simulink model "pend_dob_v"  (R2018b)
settings: Solver=VariableStepAuto  StartTime=0.0  StopTime=20  MaxStep=1e-2  RelTol=1e-3
values from neighbouring files (symbols this model uses):
  g = 9.8    [pendulo_circular.m]    (also in pendulo_doble.m; pendulo_giratorio.m)
  l1 = 0.25    [pendulo_doble.m]
  l2 = 0.5    [pendulo_doble.m]
  m1 = 0.5    [pendulo_doble.m]
  t1ini = deg2rad(10)    [pendulo_doble.m]
  t1pini = deg2rad(0)    [pendulo_doble.m]
  t2ini = deg2rad(60)    [pendulo_doble.m]
  t2pini = deg2rad(0)    [pendulo_doble.m]
settings Model: Creator=Acer  LastModifiedBy=Acer
settings DataIOCC: ReturnWorkspaceOutputs=on

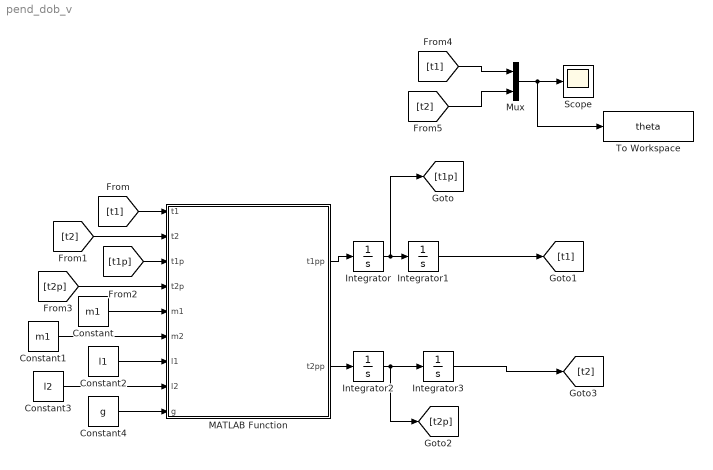
== system pend_dob_v ==
  Constant : Constant  Value=m1
  Constant1 : Constant  Value=m1
  Constant2 : Constant  Value=l1
  Constant3 : Constant  Value=l2
  Constant4 : Constant  Value=g
  Integrator : Integrator  InitialCondition=t1pini
  Integrator1 : Integrator  InitialCondition=t1ini
  Integrator2 : Integrator  InitialCondition=t2pini
  Integrator3 : Integrator  InitialCondition=t2ini
  MATLAB Function : MATLAB Function  TreatAsAtomicUnit=on
  Mux : Mux  Inputs=2
  Scope : Scope
  To Workspace : ToWorkspace  VariableName=theta  SaveFormat=Structure With Time  SampleTime=-1
  wires:
  MATLAB Function/1(t1pp) -> Integrator/1
  Integrator/1 -> [t1p], Integrator1/1
  MATLAB Function/2(t2pp) -> Integrator2/1
  Integrator2/1 -> Integrator3/1, [t2p]
  [t1] -> MATLAB Function/1(t1)
  Integrator1/1 -> [t1]
  [t2] -> MATLAB Function/2(t2)
  [t1p] -> MATLAB Function/3(t1p)
  [t2p] -> MATLAB Function/4(t2p)
  Integrator3/1 -> [t2]
  Mux/1 -> To Workspace/1, Scope/1
  [t1] -> Mux/1
  [t2] -> Mux/2
  Constant/1 -> MATLAB Function/5(m1)
  Constant1/1 -> MATLAB Function/6(m2)
  Constant2/1 -> MATLAB Function/7(l1)
  Constant3/1 -> MATLAB Function/8(l2)
  Constant4/1 -> MATLAB Function/9(g)

== matlab function pend_dob_v/MATLAB Function ==
  data: t1 input; t1pp output; t2 input; t1p input; t2p input; t2pp output; m1 input; m2 input; l1 input; l2 input; g input
function [t1pp,t2pp] = fcn(t1,t2,t1p,t2p,m1,m2,l1,l2,g)
% m1=1;
% m2=1;
% l1=1;
% l2=1;
% g=9.8;

dt=t1-t2;
mu=1+m1/m2;
m=m1/m2;

% t1pp=(g*(sin(t2)*cos(dt)-mu*sin(t1))-sin(dt)*(l2*t2p^2+l1*t1p^2*cos(dt)))/(l1*(mu-(cos(dt))^2));
% t2pp=(g*mu*(sin(t1)*cos(dt)-sin(t2))-sin(dt)*(mu*l1*t1p^2+l2*t2p^2*cos(dt)))/(l2*(mu-(cos(dt))^2));

t1pp=(cos(dt)*((g/l1)*sin(t2)-t1p^2*sin(dt))-(l2/l1)*((m+1)*(g/l2)*sin(t1)+t2p^2*sin(dt)))/(m+(sin(dt))^2);
t2pp=(cos(dt)*((m+1)*(g/l2)*sin(t1)+t2p^2*sin(dt))-(m+1)*(l1/l2)*((g/l1)*sin(t2)-t1p^2*sin(dt)))/(m+(sin(dt))^2);
